simulink model "PreLab"  (R2016a)
settings: Solver=FixedStepDiscrete  StartTime=0.0  StopTime=2000  FixedStep=1  RelTol=1e-3
libraries: hdlsllib x1
settings Model: Creator=vu.du  LastModifiedBy=duyvu
settings DataIOCC: LimitDataPoints=on  SaveFormat=Array
settings DebuggingCC: SolverPrmCheckMsg=warning
settings HardwareCC: ProdBitPerPointer=32  ProdLargestAtomicFloat=None  ProdIntDivRoundTo=Undefined  ProdEndianess=Unspecified  ProdWordSize=32  ProdHWDeviceType=32-bit Generic
settings ModelReferenceCC: PropagateSignalLabelsOutOfModel=off
settings ConfigComp: CovModelRefEnable=Off  CovSFcnEnable=off

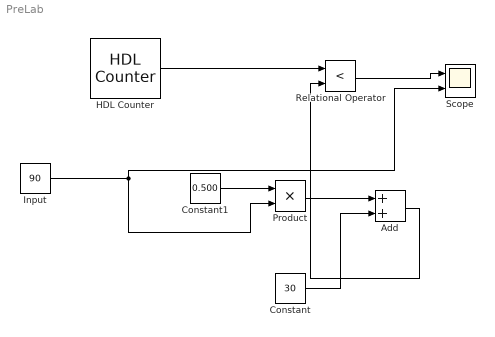
== system PreLab ==
  Add : Sum
  Constant : Constant  Value=30
  Constant1 : Constant  Value=0.500
  HDL Counter : hdlsllib/HDL Operations/HDL Counter  CountType=Count limited  CountInit=0  CountStep=1  CountMax=1000  CountFromType=Initial value  CountFrom=0  CountResetPort=off  CountLoadPort=off  CountEnbPort=off  CountDirPort=off  CountDataType=Unsigned  CountWordLen=32  CountFracLen=0  CountSampTime=1
  Input : Constant  Value=90
  Product : Product
  Relational Operator : RelationalOperator  Operator=<  OutDataTypeStr=boolean
  Scope : Scope  NumInputPorts=2
  wires:
  HDL Counter/1 -> Relational Operator/1
  Relational Operator/1 -> Scope/1
  Product/1 -> Add/1
  Constant/1 -> Add/2
  Constant1/1 -> Product/1
  Input/1 -> Scope/2, Product/2
  Add/1 -> Relational Operator/2
